simulink model "Autonomous_Driving"  (R2022a)
settings: Solver=VariableStepAuto  StartTime=0.0  StopTime=10.0  RelTol=1e-3
settings Model: Creator=udayakumar  LastModifiedBy=udayakumar

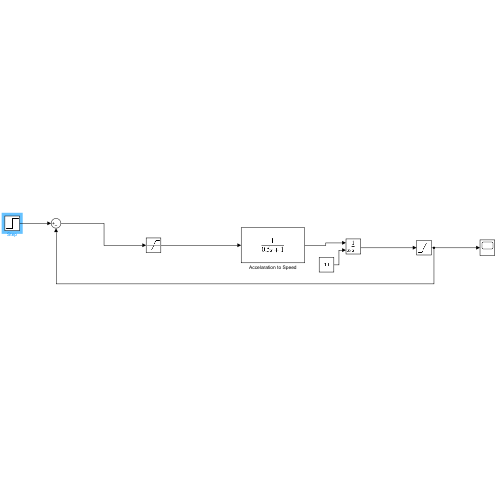
[thumbnail: Simulink's stored preview of the top-level diagram]
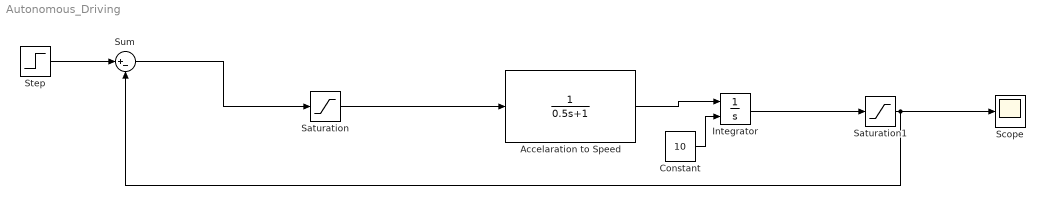
== system Autonomous_Driving ==
  Accelaration to Speed : TransferFcn  Denominator=[0.5 1]
  Constant : Constant  Value=10
  Integrator : Integrator  InitialConditionSource=external
  Saturation : Saturate  UpperLimit=2  LowerLimit=-3
  Saturation1 : Saturate  UpperLimit=inf
  Scope : Scope
  Step : Step  Time=0  Before=20  After=20  SampleTime=0
  Sum : Sum  Inputs=|+-
  wires:
  Accelaration to Speed/1 -> Integrator/1
  Constant/1 -> Integrator/2
  Step/1 -> Sum/1
  Sum/1 -> Saturation/1
  Saturation/1 -> Accelaration to Speed/1
  Integrator/1 -> Saturation1/1
  Saturation1/1 -> Sum/2, Scope/1
